simulink model "ControleIntegralTrajNominalSimulink"  (R2019a)
settings: Solver=VariableStepAuto  StartTime=0.0  StopTime=170  RelTol=1e-3
undefined symbols (not defined in the file): A, B, C, D, K, Ke
settings Model: Creator=Cliente  LastModifiedBy=Cliente

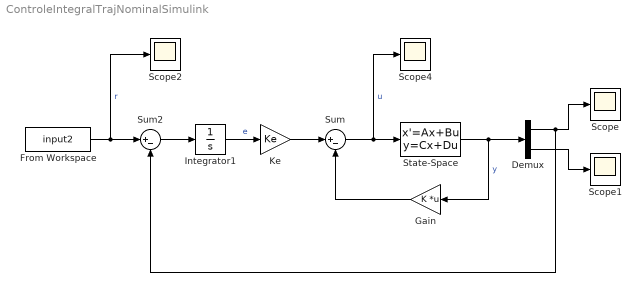
== system ControleIntegralTrajNominalSimulink ==
  Demux : Demux  Outputs=2
  From Workspace : FromWorkspace  VariableName=input2  SampleTime=0
  Gain : Gain  Gain=K  Multiplication=Matrix(K*u) (u vector)
  Integrator1 : Integrator
  Ke : Gain  Gain=Ke
  Scope{,1..2,4} (4 alike) : Scope
  State-Space : StateSpace  A=A  B=B  C=C  D=D  InitialCondition=[0; 0]
  Sum : Sum  Inputs=|+-
  Sum2 : Sum  Inputs=|+-
  wires:
  Sum/1 -> State-Space/1, Scope4/1  "u"
  Gain/1 -> Sum/2
  State-Space/1 -> Demux/1, Gain/1  "y"
  From Workspace/1 -> Scope2/1, Sum2/1  "r"
  Ke/1 -> Sum/1
  Integrator1/1 -> Ke/1  "e"
  Sum2/1 -> Integrator1/1
  Demux/2 -> Scope1/1
  Demux/1 -> Sum2/2, Scope/1
